simulink model "ControllerPID"  (R2021a)
settings: Solver=VariableStepAuto  StartTime=0.0  StopTime=5  RelTol=1e-3
values from neighbouring files (symbols this model uses):
  CF = 1300    [Data.mat]    (also in Script.m)
  i = 63    [Data.mat]
  Km = 0.0273    [Data.mat]
  Lw = 0.000103    [Data.mat]
  Rw = 0.331    [Data.mat]
  sampleTime = 0.001    [Data.mat]    (also in Script.m)
libraries: cstblocks x2, pid_lib x2
settings Model: Creator=circl  LastModifiedBy=circl
settings SolverCC: AlgebraicLoopSolver=TrustRegion

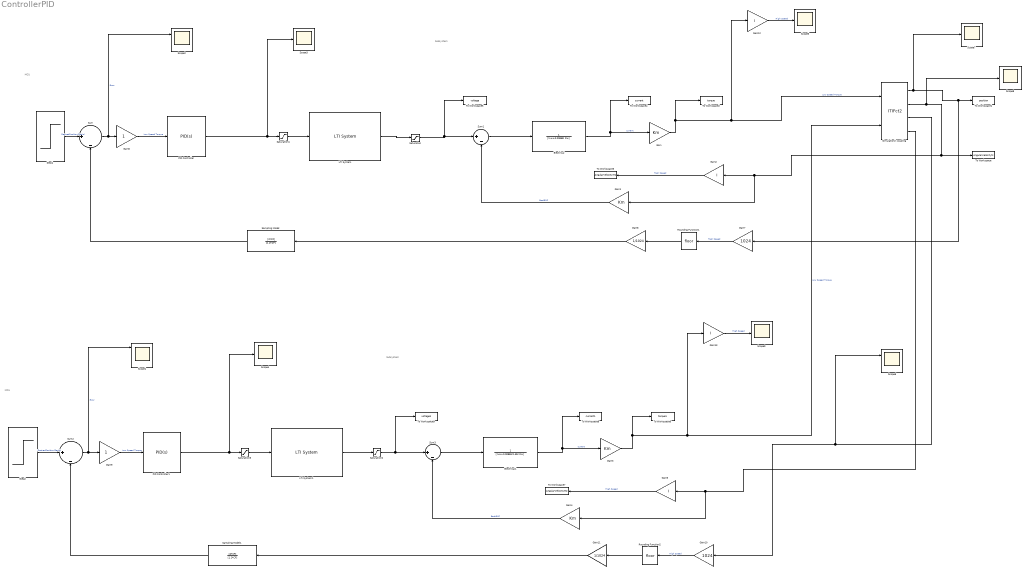
== system ControllerPID ==
  note: Subsystem
  note: MCU
  note: Subsystem
  note: MCU
  Electrical : TransferFcn  Denominator=[(Lw+0.00855) Rw]
  Electrical1 : TransferFcn  Denominator=[(Lw+0.00855*1.85) Rw]
  Gain{,1,3..4} (4 alike) : Gain  Gain=Km
  Gain10 : Gain  Gain=1024
  Gain11 : Gain  Gain=1/1024
  Gain{2,5,12..13} (4 alike) : Gain  Gain=i
  Gain6 : Gain
  Gain7 : Gain  Gain=1024
  Gain8 : Gain  Gain=1/1024
  Gain9 : Gain
  LTI System : cstblocks/LTI System  sys=AmpMotor  IC=[]
  LTI System1 : cstblocks/LTI System  sys=AmpMotor  IC=[]
  PID Controller : pid_lib/PID Controller  Controller=PID  Form=Parallel  TimeDomain=Continuous-time  UseExternalTs=off  SampleTime=-1  IntegratorMethod=Forward Euler  FilterMethod=Forward Euler  ControllerParametersSource=internal  P=0.52*3.75  I=1.875*2.45  D=0.17*1.75  UseFilter=on  N=2600  TunerSelectOption=Transfer Function Based (PID Tuner App)  InitialConditionSource=internal  InitialConditionForIntegrator=0  InitialConditionForFilter=0  DifferentiatorICPrevScaledInput=0  ExternalReset=none  TrackingMode=off  Kt=1  LimitOutput=off  SatLimitsSource=internal  UpperSaturationLimit=inf  LowerSaturationLimit=-inf  LinearizeAsGain=on  AntiWindupMode=none  Kb=1  POutMin=[]  POutMax=[]  IOutMin=[]  IOutMax=[]  DOutMin=[]  DOutMax=[]  NOutMin=[]  NOutMax=[]  SumOutMin=[]  SumOutMax=[]  SaturationOutMin=[]  SaturationOutMax=[]  PParamMin=[]  PParamMax=[]  IParamMin=[]  IParamMax=[]  DParamMin=[]  DParamMax=[]  NParamMin=[]  NParamMax=[]  KbParamMin=[]  KbParamMax=[]  KtParamMin=[]  KtParamMax=[]  KbOutMin=[]  KbOutMax=[]  KtOutMin=[]  KtOutMax=[]  IntegratorOutMin=[]  IntegratorOutMax=[]  FilterOutMin=[]  FilterOutMax=[]  SumI1OutMin=[]  SumI1OutMax=[]  SumI2OutMin=[]  SumI2OutMax=[]  SumI3OutMin=[]  SumI3OutMax=[]  SumI4OutMin=[]  SumI4OutMax=[]  SumDOutMin=[]  SumDOutMax=[]  DifferentiatorOutMin=[]  DifferentiatorOutMax=[]  FilterDiffOutCoefMin=[]  FilterDiffOutCoefMax=[]  ReciprocalOutMin=[]  ReciprocalOutMax=[]  SumDenOutMin=[]  SumDenOutMax=[]  SumNumOutMin=[]  SumNumOutMax=[]  DivideOutMin=[]  DivideOutMax=[]  UdiffTsProdOutMin=[]  UdiffTsProdOutMax=[]  NTsProdOutMin=[]  NTsProdOutMax=[]  UintegralTsProdOutMin=[]  UintegralTsProdOutMax=[]  UngainTsProdOutMin=[]  UngainTsProdOutMax=[]  IntegratorContinuousStateAttributes=''  IntegratorStateMustResolveToSignalObject=off  IntegratorRTWStateStorageClass=Auto  FilterContinuousStateAttributes=''  FilterStateMustResolveToSignalObject=off  FilterRTWStateStorageClass=Auto  ParallelPVariant=InternalParameters  IdealPVariant=Disabled  IVariant=InternalParameters  DVariant=InternalParameters  IntegratorVariant=Continuous  SatVariant=Disabled  AWVariant=Passthrough  PCopyVariant=Disabled  TRVariant=Disabled  FdbkBlocksVariant=Forward  IdealPFdbkVariant=Disabled  SatFdbkVariant=Disabled  DerivativeFilterVariant=ContFilter  NVariant=InternalParameters  NCopyVariant=Disabled  FilterICVariant=InternalICsFilter  IntegratorICVariant=InternalICs  ExternalResetVariant=Disabled  TRSumVariant=Passthrough  SumFdbkVariant=Disabled  SumVariant=Sum_PID  TsampFilterVariant=InternalTs  TsampNgainVariant=Passthrough  TsampIntegralVariant=Passthrough  ExternalSaturationOutDataTypeStr=Inherit: Same as second input
  PID Controller1 : pid_lib/PID Controller  Controller=PID  Form=Parallel  TimeDomain=Continuous-time  UseExternalTs=off  SampleTime=-1  IntegratorMethod=Forward Euler  FilterMethod=Forward Euler  ControllerParametersSource=internal  P=0.52*3.75/1.55  I=1.875*2.45/1.55  D=0.17  UseFilter=on  N=2600  TunerSelectOption=Transfer Function Based (PID Tuner App)  InitialConditionSource=internal  InitialConditionForIntegrator=0  InitialConditionForFilter=0  DifferentiatorICPrevScaledInput=0  ExternalReset=none  TrackingMode=off  Kt=1  LimitOutput=off  SatLimitsSource=internal  UpperSaturationLimit=inf  LowerSaturationLimit=-inf  LinearizeAsGain=on  AntiWindupMode=none  Kb=1  POutMin=[]  POutMax=[]  IOutMin=[]  IOutMax=[]  DOutMin=[]  DOutMax=[]  NOutMin=[]  NOutMax=[]  SumOutMin=[]  SumOutMax=[]  SaturationOutMin=[]  SaturationOutMax=[]  PParamMin=[]  PParamMax=[]  IParamMin=[]  IParamMax=[]  DParamMin=[]  DParamMax=[]  NParamMin=[]  NParamMax=[]  KbParamMin=[]  KbParamMax=[]  KtParamMin=[]  KtParamMax=[]  KbOutMin=[]  KbOutMax=[]  KtOutMin=[]  KtOutMax=[]  IntegratorOutMin=[]  IntegratorOutMax=[]  FilterOutMin=[]  FilterOutMax=[]  SumI1OutMin=[]  SumI1OutMax=[]  SumI2OutMin=[]  SumI2OutMax=[]  SumI3OutMin=[]  SumI3OutMax=[]  SumI4OutMin=[]  SumI4OutMax=[]  SumDOutMin=[]  SumDOutMax=[]  DifferentiatorOutMin=[]  DifferentiatorOutMax=[]  FilterDiffOutCoefMin=[]  FilterDiffOutCoefMax=[]  ReciprocalOutMin=[]  ReciprocalOutMax=[]  SumDenOutMin=[]  SumDenOutMax=[]  SumNumOutMin=[]  SumNumOutMax=[]  DivideOutMin=[]  DivideOutMax=[]  UdiffTsProdOutMin=[]  UdiffTsProdOutMax=[]  NTsProdOutMin=[]  NTsProdOutMax=[]  UintegralTsProdOutMin=[]  UintegralTsProdOutMax=[]  UngainTsProdOutMin=[]  UngainTsProdOutMax=[]  IntegratorContinuousStateAttributes=''  IntegratorStateMustResolveToSignalObject=off  IntegratorRTWStateStorageClass=Auto  FilterContinuousStateAttributes=''  FilterStateMustResolveToSignalObject=off  FilterRTWStateStorageClass=Auto  ParallelPVariant=InternalParameters  IdealPVariant=Disabled  IVariant=InternalParameters  DVariant=InternalParameters  IntegratorVariant=Continuous  SatVariant=Disabled  AWVariant=Passthrough  PCopyVariant=Disabled  TRVariant=Disabled  FdbkBlocksVariant=Forward  IdealPFdbkVariant=Disabled  SatFdbkVariant=Disabled  DerivativeFilterVariant=ContFilter  NVariant=InternalParameters  NCopyVariant=Disabled  FilterICVariant=InternalICsFilter  IntegratorICVariant=InternalICs  ExternalResetVariant=Disabled  TRSumVariant=Passthrough  SumFdbkVariant=Disabled  SumVariant=Sum_PID  TsampFilterVariant=InternalTs  TsampNgainVariant=Passthrough  TsampIntegralVariant=Passthrough  ExternalSaturationOutDataTypeStr=Inherit: Same as second input
  Rounding Function1 : Rounding
  Rounding Function2 : Rounding
  Sampling Model : TransferFcn  Numerator=[2*CF]  Denominator=[1 2*CF]
  Sampling Model1 : TransferFcn  Numerator=[2*CF]  Denominator=[1 2*CF]
  Saturation : Saturate  UpperLimit=24  LowerLimit=-24
  Saturation1 : Saturate  UpperLimit=5  LowerLimit=-5
  Saturation2 : Saturate  UpperLimit=24  LowerLimit=-24
  Saturation3 : Saturate  UpperLimit=5  LowerLimit=-5
  Scope1 : Scope  NumInputPorts=3
  Scope2 : Scope  NumInputPorts=2
  Scope{3..5,7..9} (6 alike) : Scope
  Scope6 : Scope  NumInputPorts=2
  SimulationX coupling : S-Function  FunctionName=ITIFct2  Parameters=ip, port, ts, nIn, nOut  SFunctionDeploymentMode=off  EnableBusSupport=off  mask{ip='localhost', port=4097, ts=0.001, nIn=2, nOut=4}
      mask prompts: ip "Address: ip"; port "Port Number: port [-]"; ts "Communication Step Size: ts [s]"; nIn "Input Vector Dimension (to SimulationX): nIn [-]"; nOut "Output Vector Dimension (from SimulationX): nOut [-]"
      mask help: Coupling Element
  Step1 : Step  Time=2.5  Before=pi/2  After=0  SampleTime=sampleTime
  Step2 : Step  Time=2.5  Before=-pi/2  After=0  SampleTime=sampleTime
  Sum{,1..3} (4 alike) : Sum  Inputs=|+-
  To Workspace : ToWorkspace  VariableName=AngularVelocityM  SaveFormat=Timeseries  SampleTime=sampleTime
  To Workspace1 : ToWorkspace  VariableName=position  SaveFormat=Timeseries  SampleTime=-1
  To Workspace2 : ToWorkspace  VariableName=torque  SaveFormat=Timeseries  SampleTime=-1
  To Workspace3 : ToWorkspace  VariableName=AngularVelocityM1  SaveFormat=Timeseries  SampleTime=sampleTime
  To Workspace4 : ToWorkspace  VariableName=current  SaveFormat=Timeseries  SampleTime=-1
  To Workspace5 : ToWorkspace  VariableName=voltage  SaveFormat=Timeseries  SampleTime=-1
  To Workspace6 : ToWorkspace  VariableName=torque1  SaveFormat=Timeseries  SampleTime=-1
  To Workspace7 : ToWorkspace  VariableName=AngularVelocityM2  SaveFormat=Timeseries  SampleTime=sampleTime
  To Workspace8 : ToWorkspace  VariableName=current1  SaveFormat=Timeseries  SampleTime=-1
  To Workspace9 : ToWorkspace  VariableName=voltage1  SaveFormat=Timeseries  SampleTime=-1
  wires:
  Step1/1 -> Sum/1  "DesiredPosition(Rad/s)"
  Gain2/1 -> To Workspace3/1  "High Speed"
  Gain/1 -> To Workspace2/1, Gain12/1, SimulationX coupling/1  "Low Speed Torque"
  Gain1/1 -> Sum1/2  "BackEMF"
  Sum1/1 -> Electrical/1
  Electrical/1 -> To Workspace4/1, Gain/1  "current"
  Sampling Model/1 -> Sum/2
  Sum/1 -> Gain6/1, Scope2/1  "Error"
  SimulationX coupling/2 -> Scope8/1, Gain1/1, Gain2/1, To Workspace/1
  LTI System/1 -> Saturation/1
  Saturation/1 -> To Workspace5/1, Sum1/1
  SimulationX coupling/1 -> Scope7/1, Gain7/1, To Workspace1/1
  Gain6/1 -> PID Controller/1  "Low Speed Torque"
  Gain8/1 -> Sampling Model/1
  Rounding Function1/1 -> Gain8/1
  Gain7/1 -> Rounding Function1/1  "High Speed"
  PID Controller/1 -> Saturation1/1, Scope3/1
  Saturation1/1 -> LTI System/1
  Saturation3/1 -> LTI System1/1
  Gain10/1 -> Rounding Function2/1  "High Speed"
  Rounding Function2/1 -> Gain11/1
  Gain9/1 -> PID Controller1/1  "Low Speed Torque"
  Saturation2/1 -> To Workspace9/1, Sum3/1
  SimulationX coupling/3 -> Gain10/1, Scope6/1
  SimulationX coupling/4 -> Gain4/1, Gain5/1
  LTI System1/1 -> Saturation2/1
  Gain11/1 -> Sampling Model1/1
  Electrical1/1 -> To Workspace8/1, Gain3/1  "current"
  Sum2/1 -> Gain9/1, Scope1/1  "Error"
  Sum3/1 -> Electrical1/1
  Gain4/1 -> Sum3/2  "BackEMF"
  PID Controller1/1 -> Scope4/1, Saturation3/1
  Sampling Model1/1 -> Sum2/2
  Step2/1 -> Sum2/1  "DesiredPosition(Rad/s)"
  Gain5/1 -> To Workspace7/1  "High Speed"
  Gain12/1 -> Scope5/1  "High Speed"
  Gain13/1 -> Scope9/1  "High Speed"
  Gain3/1 -> Gain13/1, SimulationX coupling/2, To Workspace6/1  "Low Speed Torque"
